simulink model "SR_SNN"  (R2022a)
settings: Solver=ode15s  StartTime=0.0  StopTime=NTimeSteps  RelTol=1e-3
values from neighbouring files (symbols this model uses):
  Etol = 10    [SR_Main_Script_Sim.m]
  t_iterO = 1    [SR_Main_Script_Sim.m]
  Ts = 1    [SR_Main_Script_Sim.m]
  Tx = 1    [SR_Main_Script_Sim.m]
  Txi = r*cos(xx)    [SR_Main_Script_Sim.m]
  Ty = 1    [SR_Main_Script_Sim.m]
  Tyi = r*sin(yy)    [SR_Main_Script_Sim.m]
  Tz = 2    [SR_Main_Script_Sim.m]
  x_i = [[1] ... (first row only)    [SR_Main_Script_Sim.m]
libraries: slpidlib x3, cstblocks x3, dspnetwork x2
settings Model: Creator=Pouya  LastModifiedBy=Pouya
settings DebuggingCC: UnconnectedInputMsg=warning  UnconnectedOutputMsg=warning  UnconnectedLineMsg=warning
settings RTWCC: DLArmComputeVersion=19.05

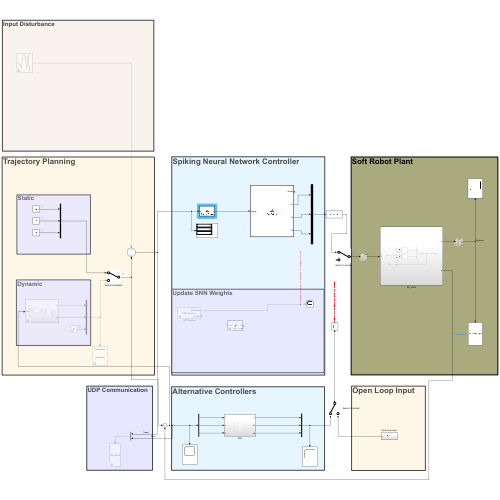
[thumbnail: Simulink's stored preview of the top-level diagram]
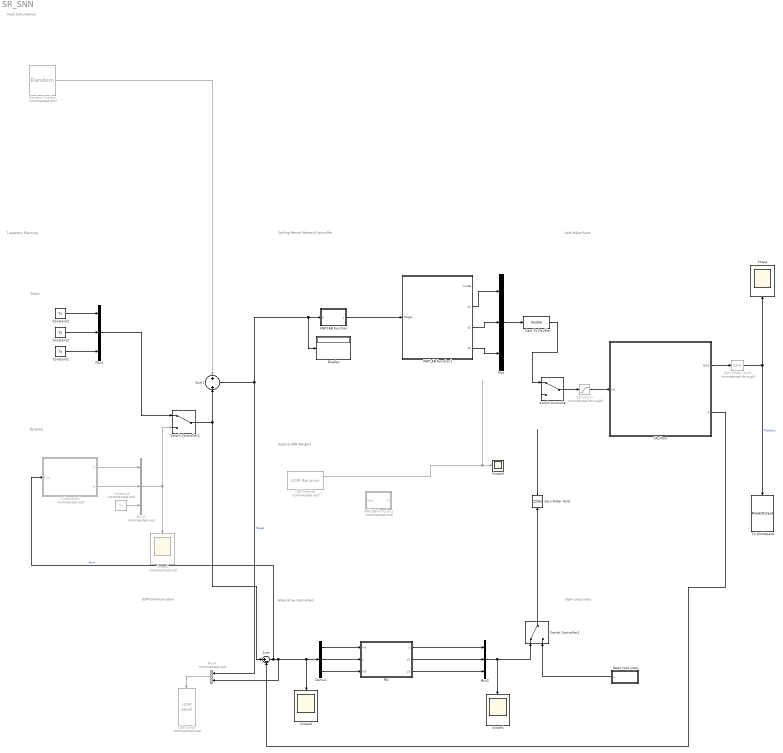
== system SR_SNN ==
  note: UDP Communication
  note: Update SNN Weights
  note: Input Disturbance
  note: Dynamic
  note: Static
  note: Open Loop Input
  note: Alternative Controllers
  note: Trajectory Planning
  note: Soft Robot Plant
  note: Spiking Neural Network Controller
  Cast To Double : DataTypeConversion  OutDataTypeStr=double  SaturateOnIntegerOverflow=off  RndMeth=Floor
  Constant1 : Constant  Value=Tz
  Constant2 : Constant  Value=Tx
  Constant3 : Constant  Value=Ty
  Constant4 : Constant  Commented=on  Value=Tz
  Demux : Demux  Outputs=3
  Display : Display
  MATLAB Function : MATLAB Function  TreatAsAtomicUnit=on
  MATLAB Function1 : MATLAB Function  TreatAsAtomicUnit=on
  MATLAB Function2 : MATLAB Function  Commented=on  TreatAsAtomicUnit=on
  Mux : Mux  Inputs=3
  Mux1 : Mux  Inputs=3
  Mux2 : Mux  Inputs=3
  Mux3 : Mux  Commented=on  Inputs=3
  Mux4 : Mux  Commented=on  Inputs=2
  Open loop input : Subsystem
  PID : Subsystem
  Random Number : RandomNumber  Commented=on  SampleTime=0.1
  SR_Plant : Subsystem
  Saturation : Saturate  Commented=through  UpperLimit=4  LowerLimit=-4
  Scope{,1,3..4} (4 alike) : Scope
  Scope2 : Scope  Commented=on
  Subsystem1 : Subsystem  Commented=on
  Sum : Sum  Inputs=|+-
  Sum1 : Sum
  Switch Controller : ManualSwitch
  Switch Controller1 : ManualSwitch
  Switch Controller2 : ManualSwitch
  To Workspace : ToWorkspace  VariableName=ModelOutput  SaveFormat=Timeseries  SampleTime=-1
  UDP Receive : dspnetwork/UDP Receive  Commented=on  localURL='0.0.0.0'  localPort=54320  remoteURL='127.0.0.1'  remotePort=-1  recvBufferSize=1024  dims=1  signalDatatype=uint8  isComplex=off  isVarSize=off  showBlockingTime=off  blockingTime=0  sampletime=1  blockPlatform=[]
  UDP Send1 : dspnetwork/UDP Send  Commented=on  remoteURL='127.0.0.1'  remotePort=54320  localURL='0.0.0.0'  localPortSource=Automatically determine  localPort=54320  sendBufferSize=1024  sampletime=-1  blockPlatform=[]  separateLengthPort=0
  Zero-Order Hold : ZeroOrderHold  SampleTime=Ts
  Zero-Order Hold1 : ZeroOrderHold  Commented=through  SampleTime=Ts
  wires:
  Constant2/1 -> Mux1/1
  Constant3/1 -> Mux1/2
  SR_Plant/1(Out1) -> Zero-Order Hold1/1
  SR_Plant/2(p) -> Sum/2
  Switch Controller/1 -> Saturation/1
  Constant1/1 -> Mux1/3
  Switch Controller1/1 -> Zero-Order Hold/1
  Open loop input/1(u) -> Switch Controller1/2
  Zero-Order Hold/1 -> ?
  Demux/2 -> PID/2(u)
  Demux/1 -> PID/1(In1)
  Demux/3 -> PID/3(In3)
  PID/1(y) -> Mux2/1
  Saturation/1 -> SR_Plant/1(In1)
  PID/2(y1) -> Mux2/2
  PID/3(y2) -> Mux2/3
  Mux2/1 -> Switch Controller1/1, Scope1/1
  Switch Controller2/1 -> Sum/1, Sum1/2
  Mux1/1 -> Switch Controller2/1
  Mux3/1 -> Switch Controller2/2, Scope2/1
  Subsystem1/2(Ty) -> Mux3/2
  Subsystem1/1(Tx) -> Mux3/1
  Constant4/1 -> Mux3/3
  MATLAB Function1/2(s1) -> Mux/1
  MATLAB Function1/3(s2) -> Mux/2
  MATLAB Function1/4(s3) -> Mux/3
  Sum/1 -> Scope3/1, Demux/1, Mux4/2, Subsystem1/1(Error)  "Error"
  Zero-Order Hold1/1 -> Scope/1, To Workspace/1  "Positions"
  UDP Receive/1 -> Scope4/1
  Random Number/1 -> Sum1/1
  Sum1/1 -> Display/1, MATLAB Function/1(u), Mux4/1  "Target"
  Mux4/1 -> UDP Send1/1
  MATLAB Function/1(y) -> MATLAB Function1/1(Target)
  Mux/1 -> Cast To Double/1
  Cast To Double/1 -> Switch Controller/1

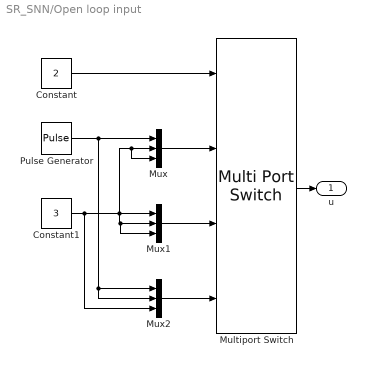
== system SR_SNN/Open loop input ==
  Constant : Constant  Value=2
  Constant1 : Constant  Value=3
  Multiport Switch : MultiPortSwitch  SaturateOnIntegerOverflow=off  InputSameDT=off
  Mux : Mux  Inputs=3
  Mux1 : Mux  Inputs=3
  Mux2 : Mux  Inputs=3
  Pulse Generator : DiscretePulseGenerator  PulseType=Time based  Period=5  PulseWidth=10
  u : Outport
  wires:
  Constant1/1 -> Mux2/3, Mux1/3, Mux1/2, Mux1/1, Mux/3, Mux/2
  Pulse Generator/1 -> Mux2/2, Mux2/1, Mux/1
  Constant/1 -> Multiport Switch/1
  Mux2/1 -> Multiport Switch/4
  Mux/1 -> Multiport Switch/2
  Multiport Switch/1 -> u/1
  Mux1/1 -> Multiport Switch/3

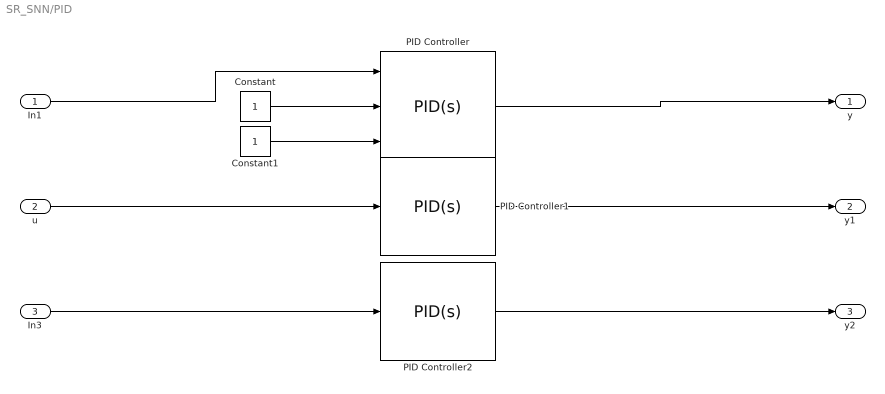
== system SR_SNN/PID ==
  In1 : Inport
  u : Inport  Port=2
  In3 : Inport  Port=3
  Constant : Constant
  Constant1 : Constant
  PID Controller : slpidlib/PID Controller  Controller=PID  Form=Parallel  TimeDomain=Continuous-time  UseExternalTs=off  SampleTime=-1  IntegratorMethod=Forward Euler  FilterMethod=Forward Euler  ControllerParametersSource=internal  P=-0.00389726842961966  I=-9.20575835453352e-05  UseKiTs=off  D=-0.0366591203292117  N=462.720758480725  UseFilter=on  TunerSelectOption=Transfer Function Based (PID Tuner App)  InitialConditionSource=external  InitialConditionForIntegrator=0  InitialConditionForFilter=0  DifferentiatorICPrevScaledInput=0  ExternalReset=none  TrackingMode=off  Kt=1  LimitOutput=off  SatLimitsSource=internal  UpperSaturationLimit=inf  LowerSaturationLimit=-inf  LinearizeAsGain=on  AntiWindupMode=none  Kb=1  POutMin=[]  POutMax=[]  IOutMin=[]  IOutMax=[]  DOutMin=[]  DOutMax=[]  NOutMin=[]  NOutMax=[]  SumOutMin=[]  SumOutMax=[]  SaturationOutMin=[]  SaturationOutMax=[]  PParamMin=[]  PParamMax=[]  IParamMin=[]  IParamMax=[]  DParamMin=[]  DParamMax=[]  NParamMin=[]  NParamMax=[]  KbParamMin=[]  KbParamMax=[]  KtParamMin=[]  KtParamMax=[]  KbOutMin=[]  KbOutMax=[]  KtOutMin=[]  KtOutMax=[]  IntegratorOutMin=[]  IntegratorOutMax=[]  FilterOutMin=[]  FilterOutMax=[]  SumI1OutMin=[]  SumI1OutMax=[]  SumI2OutMin=[]  SumI2OutMax=[]  SumI3OutMin=[]  SumI3OutMax=[]  SumI4OutMin=[]  SumI4OutMax=[]  SumDOutMin=[]  SumDOutMax=[]  DifferentiatorOutMin=[]  DifferentiatorOutMax=[]  FilterDiffOutCoefMin=[]  FilterDiffOutCoefMax=[]  ReciprocalOutMin=[]  ReciprocalOutMax=[]  SumDenOutMin=[]  SumDenOutMax=[]  SumNumOutMin=[]  SumNumOutMax=[]  DivideOutMin=[]  DivideOutMax=[]  UdiffTsProdOutMin=[]  UdiffTsProdOutMax=[]  NTsProdOutMin=[]  NTsProdOutMax=[]  UintegralTsProdOutMin=[]  UintegralTsProdOutMax=[]  UngainTsProdOutMin=[]  UngainTsProdOutMax=[]  IntegratorContinuousStateAttributes=''  IntegratorStateMustResolveToSignalObject=off  IntegratorRTWStateStorageClass=Auto  FilterContinuousStateAttributes=''  FilterStateMustResolveToSignalObject=off  FilterRTWStateStorageClass=Auto  ParallelPVariant=InternalParameters  IdealPVariant=Disabled  IVariant=InternalParameters  DVariant=InternalParameters  IntegratorVariant=Continuous  SatVariant=Disabled  AWVariant=Passthrough  PCopyVariant=Disabled  TRVariant=Disabled  FdbkBlocksVariant=Forward  IdealPFdbkVariant=Disabled  SatFdbkVariant=Disabled  DerivativeFilterVariant=ContFilter  NVariant=InternalParameters  NCopyVariant=Disabled  FilterICVariant=ExternalICs  IntegratorICVariant=ExternalICs  ExternalResetVariant=Disabled  TRSumVariant=Passthrough  SumFdbkVariant=Disabled  SumVariant=Sum_PID  TsampFilterVariant=InternalTs  TsampNgainVariant=Passthrough  TsampIntegralVariant=Passthrough  ExternalSaturationOutDataTypeStr=Inherit: Same as second input  aMode=0
  PID Controller1 : slpidlib/PID Controller  Controller=PID  Form=Parallel  TimeDomain=Continuous-time  UseExternalTs=off  SampleTime=-1  IntegratorMethod=Forward Euler  FilterMethod=Forward Euler  ControllerParametersSource=internal  P=0.79056648520257  I=12.0335076656055  UseKiTs=off  D=0.00902589117456867  N=93.9877255340492  UseFilter=on  TunerSelectOption=Transfer Function Based (PID Tuner App)  InitialConditionSource=internal  InitialConditionForIntegrator=0  InitialConditionForFilter=0  DifferentiatorICPrevScaledInput=0  ExternalReset=none  TrackingMode=off  Kt=1  LimitOutput=off  SatLimitsSource=internal  UpperSaturationLimit=inf  LowerSaturationLimit=-inf  LinearizeAsGain=on  AntiWindupMode=none  Kb=1  POutMin=[]  POutMax=[]  IOutMin=[]  IOutMax=[]  DOutMin=[]  DOutMax=[]  NOutMin=[]  NOutMax=[]  SumOutMin=[]  SumOutMax=[]  SaturationOutMin=[]  SaturationOutMax=[]  PParamMin=[]  PParamMax=[]  IParamMin=[]  IParamMax=[]  DParamMin=[]  DParamMax=[]  NParamMin=[]  NParamMax=[]  KbParamMin=[]  KbParamMax=[]  KtParamMin=[]  KtParamMax=[]  KbOutMin=[]  KbOutMax=[]  KtOutMin=[]  KtOutMax=[]  IntegratorOutMin=[]  IntegratorOutMax=[]  FilterOutMin=[]  FilterOutMax=[]  SumI1OutMin=[]  SumI1OutMax=[]  SumI2OutMin=[]  SumI2OutMax=[]  SumI3OutMin=[]  SumI3OutMax=[]  SumI4OutMin=[]  SumI4OutMax=[]  SumDOutMin=[]  SumDOutMax=[]  DifferentiatorOutMin=[]  DifferentiatorOutMax=[]  FilterDiffOutCoefMin=[]  FilterDiffOutCoefMax=[]  ReciprocalOutMin=[]  ReciprocalOutMax=[]  SumDenOutMin=[]  SumDenOutMax=[]  SumNumOutMin=[]  SumNumOutMax=[]  DivideOutMin=[]  DivideOutMax=[]  UdiffTsProdOutMin=[]  UdiffTsProdOutMax=[]  NTsProdOutMin=[]  NTsProdOutMax=[]  UintegralTsProdOutMin=[]  UintegralTsProdOutMax=[]  UngainTsProdOutMin=[]  UngainTsProdOutMax=[]  IntegratorContinuousStateAttributes=''  IntegratorStateMustResolveToSignalObject=off  IntegratorRTWStateStorageClass=Auto  FilterContinuousStateAttributes=''  FilterStateMustResolveToSignalObject=off  FilterRTWStateStorageClass=Auto  ParallelPVariant=InternalParameters  IdealPVariant=Disabled  IVariant=InternalParameters  DVariant=InternalParameters  IntegratorVariant=Continuous  SatVariant=Disabled  AWVariant=Passthrough  PCopyVariant=Disabled  TRVariant=Disabled  FdbkBlocksVariant=Forward  IdealPFdbkVariant=Disabled  SatFdbkVariant=Disabled  DerivativeFilterVariant=ContFilter  NVariant=InternalParameters  NCopyVariant=Disabled  FilterICVariant=InternalICsFilter  IntegratorICVariant=InternalICs  ExternalResetVariant=Disabled  TRSumVariant=Passthrough  SumFdbkVariant=Disabled  SumVariant=Sum_PID  TsampFilterVariant=InternalTs  TsampNgainVariant=Passthrough  TsampIntegralVariant=Passthrough  ExternalSaturationOutDataTypeStr=Inherit: Same as second input  aMode=0
  PID Controller2 : slpidlib/PID Controller  Controller=PID  Form=Parallel  TimeDomain=Continuous-time  UseExternalTs=off  SampleTime=-1  IntegratorMethod=Forward Euler  FilterMethod=Forward Euler  ControllerParametersSource=internal  P=0.559243071667532  I=12.7287987560963  UseKiTs=off  D=0  N=100  UseFilter=on  TunerSelectOption=Transfer Function Based (PID Tuner App)  InitialConditionSource=internal  InitialConditionForIntegrator=0  InitialConditionForFilter=0  DifferentiatorICPrevScaledInput=0  ExternalReset=none  TrackingMode=off  Kt=1  LimitOutput=off  SatLimitsSource=internal  UpperSaturationLimit=inf  LowerSaturationLimit=-inf  LinearizeAsGain=on  AntiWindupMode=none  Kb=1  POutMin=[]  POutMax=[]  IOutMin=[]  IOutMax=[]  DOutMin=[]  DOutMax=[]  NOutMin=[]  NOutMax=[]  SumOutMin=[]  SumOutMax=[]  SaturationOutMin=[]  SaturationOutMax=[]  PParamMin=[]  PParamMax=[]  IParamMin=[]  IParamMax=[]  DParamMin=[]  DParamMax=[]  NParamMin=[]  NParamMax=[]  KbParamMin=[]  KbParamMax=[]  KtParamMin=[]  KtParamMax=[]  KbOutMin=[]  KbOutMax=[]  KtOutMin=[]  KtOutMax=[]  IntegratorOutMin=[]  IntegratorOutMax=[]  FilterOutMin=[]  FilterOutMax=[]  SumI1OutMin=[]  SumI1OutMax=[]  SumI2OutMin=[]  SumI2OutMax=[]  SumI3OutMin=[]  SumI3OutMax=[]  SumI4OutMin=[]  SumI4OutMax=[]  SumDOutMin=[]  SumDOutMax=[]  DifferentiatorOutMin=[]  DifferentiatorOutMax=[]  FilterDiffOutCoefMin=[]  FilterDiffOutCoefMax=[]  ReciprocalOutMin=[]  ReciprocalOutMax=[]  SumDenOutMin=[]  SumDenOutMax=[]  SumNumOutMin=[]  SumNumOutMax=[]  DivideOutMin=[]  DivideOutMax=[]  UdiffTsProdOutMin=[]  UdiffTsProdOutMax=[]  NTsProdOutMin=[]  NTsProdOutMax=[]  UintegralTsProdOutMin=[]  UintegralTsProdOutMax=[]  UngainTsProdOutMin=[]  UngainTsProdOutMax=[]  IntegratorContinuousStateAttributes=''  IntegratorStateMustResolveToSignalObject=off  IntegratorRTWStateStorageClass=Auto  FilterContinuousStateAttributes=''  FilterStateMustResolveToSignalObject=off  FilterRTWStateStorageClass=Auto  ParallelPVariant=InternalParameters  IdealPVariant=Disabled  IVariant=InternalParameters  DVariant=InternalParameters  IntegratorVariant=Continuous  SatVariant=Disabled  AWVariant=Passthrough  PCopyVariant=Disabled  TRVariant=Disabled  FdbkBlocksVariant=Forward  IdealPFdbkVariant=Disabled  SatFdbkVariant=Disabled  DerivativeFilterVariant=ContFilter  NVariant=InternalParameters  NCopyVariant=Disabled  FilterICVariant=InternalICsFilter  IntegratorICVariant=InternalICs  ExternalResetVariant=Disabled  TRSumVariant=Passthrough  SumFdbkVariant=Disabled  SumVariant=Sum_PID  TsampFilterVariant=InternalTs  TsampNgainVariant=Passthrough  TsampIntegralVariant=Passthrough  ExternalSaturationOutDataTypeStr=Inherit: Same as second input  aMode=0
  y : Outport
  y1 : Outport  Port=2
  y2 : Outport  Port=3
  wires:
  u/1 -> PID Controller1/1
  PID Controller/1 -> y/1
  In1/1 -> PID Controller/1
  PID Controller1/1 -> y1/1
  In3/1 -> PID Controller2/1
  PID Controller2/1 -> y2/1
  Constant/1 -> PID Controller/2
  Constant1/1 -> PID Controller/3

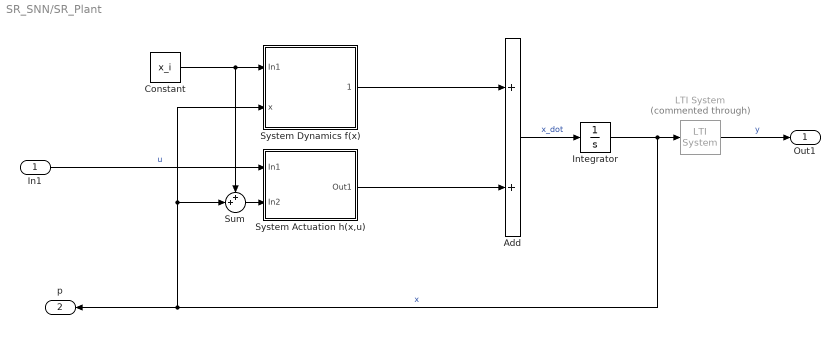
== system SR_SNN/SR_Plant ==
  In1 : Inport
  Add : Sum
  Constant : Constant  Value=x_i
  Integrator : Integrator
  LTI System : cstblocks/LTI System  Commented=through  sys=C  IC=[]
  Sum : Sum  Inputs=++|
  System Actuation h(x,u) : Subsystem
  System Dynamics f(x) : Subsystem
  Out1 : Outport
  p : Outport  Port=2
  wires:
  In1/1 -> System Actuation h(x,u)/1(In1)  "u"
  System Dynamics f(x)/1(1) -> Add/1
  System Actuation h(x,u)/1(Out1) -> Add/2
  Add/1 -> Integrator/1  "x_dot"
  Constant/1 -> Sum/1, System Dynamics f(x)/1(In1)
  Integrator/1 -> System Dynamics f(x)/2(x), Sum/2, p/1, LTI System/1  "x"
  LTI System/1 -> Out1/1  "y"
  Sum/1 -> System Actuation h(x,u)/2(In2)

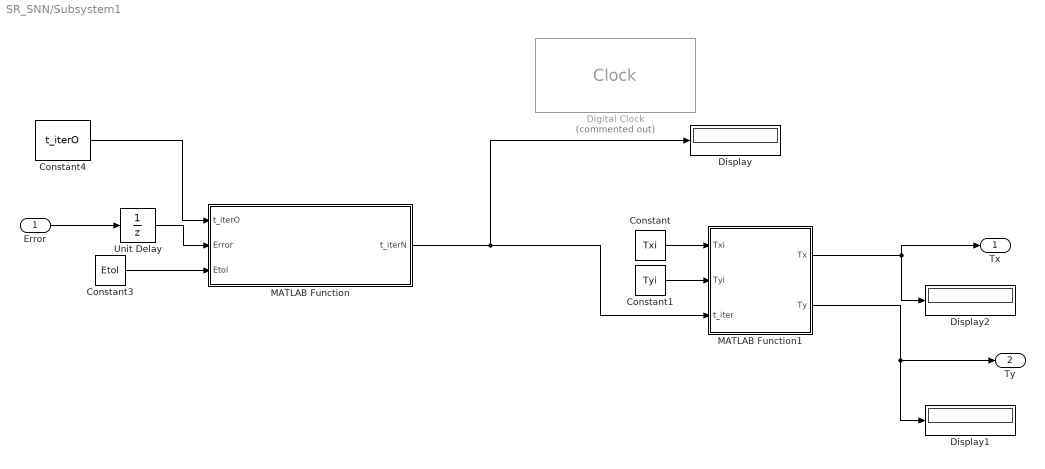
== system SR_SNN/Subsystem1 ==
  Error : Inport
  Constant : Constant  Value=Txi
  Constant1 : Constant  Value=Tyi
  Constant3 : Constant  Value=Etol
  Constant4 : Constant  Value=t_iterO
  Digital Clock : DigitalClock  Commented=on
  Display : Display
  Display1 : Display
  Display2 : Display
  MATLAB Function : MATLAB Function  TreatAsAtomicUnit=on
  MATLAB Function1 : MATLAB Function  TreatAsAtomicUnit=on
  Unit Delay : UnitDelay  SampleTime=-1  HasFrameUpgradeWarning=on
  Tx : Outport
  Ty : Outport  Port=2
  wires:
  MATLAB Function1/1(Tx) -> Tx/1, Display2/1
  MATLAB Function1/2(Ty) -> Display1/1, Ty/1
  Error/1 -> Unit Delay/1
  Constant3/1 -> MATLAB Function/3(Etol)
  MATLAB Function/1(t_iterN) -> Display/1, MATLAB Function1/3(t_iter)
  Unit Delay/1 -> MATLAB Function/2(Error)
  Constant4/1 -> MATLAB Function/1(t_iterO)
  Constant1/1 -> MATLAB Function1/2(Tyi)
  Constant/1 -> MATLAB Function1/1(Txi)

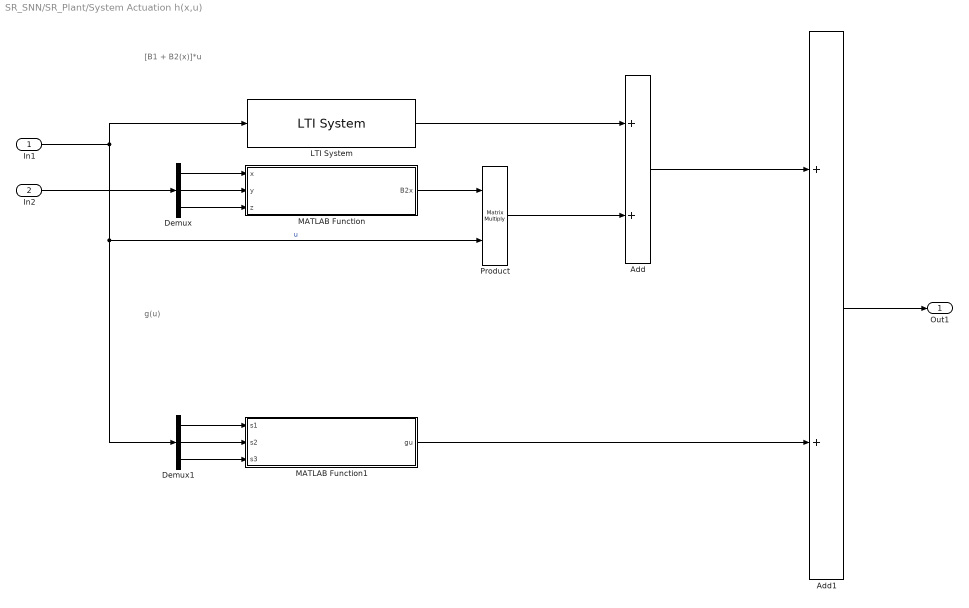
== system SR_SNN/SR_Plant/System Actuation h(x,u) ==
  note: g(u)
  note: [B1 + B2(x)]*u
  In1 : Inport
  In2 : Inport  Port=2
  Add : Sum
  Add1 : Sum
  Demux : Demux  Outputs=3
  Demux1 : Demux  Outputs=3
  LTI System : cstblocks/LTI System  sys=B1  IC=[]
  MATLAB Function : MATLAB Function  TreatAsAtomicUnit=on
  MATLAB Function1 : MATLAB Function  TreatAsAtomicUnit=on
  Product : Product  Multiplication=Matrix(*)
  Out1 : Outport
  wires:
  In1/1 -> LTI System/1, Demux1/1, Product/2  "u"
  MATLAB Function1/1(gu) -> Add1/2
  LTI System/1 -> Add/1
  Product/1 -> Add/2
  Add/1 -> Add1/1
  MATLAB Function/1(B2x) -> Product/1
  Add1/1 -> Out1/1
  In2/1 -> Demux/1
  Demux/2 -> MATLAB Function/2(y)
  Demux/1 -> MATLAB Function/1(x)
  Demux/3 -> MATLAB Function/3(z)
  Demux1/2 -> MATLAB Function1/2(s2)
  Demux1/1 -> MATLAB Function1/1(s1)
  Demux1/3 -> MATLAB Function1/3(s3)

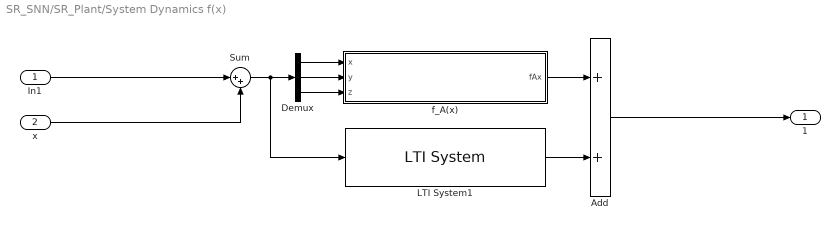
== system SR_SNN/SR_Plant/System Dynamics f(x) ==
  In1 : Inport
  x : Inport  Port=2
  Add : Sum
  Demux : Demux  Outputs=3
  LTI System1 : cstblocks/LTI System  sys=A  IC=[]
  Sum : Sum  Inputs=|++
  f_A(x) : MATLAB Function  TreatAsAtomicUnit=on
  1 : Outport
  wires:
  In1/1 -> Sum/1
  Sum/1 -> LTI System1/1, Demux/1
  Add/1 -> 1/1
  LTI System1/1 -> Add/2
  f_A(x)/1(fAx) -> Add/1
  Demux/1 -> f_A(x)/1(x)
  Demux/2 -> f_A(x)/2(y)
  Demux/3 -> f_A(x)/3(z)
  x/1 -> Sum/2

== matlab function SR_SNN/MATLAB Function1 ==
  data: model output; s1 output; s2 output; s3 output; Target input
 function [model,s1,s2,s3] = RunPython(Target)
    model=0;s1=0;s2=0;s3=0;% Has to be preassigned, otherwise Simulink throws an error
    coder.extrinsic('py.SNN_model.Run_model') % Python functions have to be run extrinsically, meaning no C code generated
    [model,s1,s2,s3] = py.SNN_model.Run_model(Target);
    
end

== matlab function SR_SNN/SR_Plant/System Dynamics f(x)/f_A(x) ==
  data: x input; fAx output; y input; z input
function fAx = f_A(x,y,z)

fAx = 10e-3*[[0.17*x^2 - 1.22*y^2 - 0.145*z^2 + 4.92*x*y + 20.3*x*z + 0.748*y*z]
           [3.39*x^2 - 1.94*y^2 + 3.48*z^2 - 1.68*x*y + 5.63*x*z + 17.0*y*z]
           [0.456*x^2 + 0.672*y^2 + 19.4*z^2 - 1.92*x*y + 1.3*x*z - 0.0985*y*z]];

== matlab function SR_SNN/SR_Plant/System Actuation h(x,u)/MATLAB Function ==
  data: x input; B2x output; y input; z input
function B2x = B2(x,y,z)

B2x = 10e-3*[[-2.86*x + 2.34*y + 16.8*z, -2.56*x - 1.23*y - 20.2*z, 1.59*x - 1.16*y + 3.61*z]
             [2.76*x + 0.356*y - 9.28*z, -2.98*x + 3.22*y - 12.9*z, -0.129*x - 4.02*y + 19.9*z]
             [-4.72*x + 3.42*y + 2.26*z, 5.47*x + 3.28*y + 1.58*z, -1.06*x - 6.62*y + 4.49*z]];

== matlab function SR_SNN/SR_Plant/System Actuation h(x,u)/MATLAB Function1 ==
  data: s1 input; gu output; s2 input; s3 input
function gu = g(s1,s2,s3)

gu = 10e-4*[[14.1*s1^2 - 8.48*s2^2 + 5.9*s3^2 - 5.02*s1*s2 - 6.56*s1*s3 + 3.04*s2*s3]
            [11.3*s1^2 - 4.67*s2^2 + 19.5*s3^2 + 1.54*s1*s2 + 3.15*s1*s3 - 1.25*s2*s3]
            [1.05*s1^2 + 2.26*s2^2 + 2.83*s3^2 - 10.6*s1*s2 - 3.2*s1*s3 - 12.7*s2*s3]];

== matlab function SR_SNN/MATLAB Function ==
  data: u input; y output
function y = ConvertDtype(u)

y = 0;
coder.extrinsic('Mat2Py')
y = Mat2Py(u);

== matlab function SR_SNN/Subsystem1/MATLAB Function ==
  data: t_iterO input; Error input; t_iterN output; Etol input
function t_iterN = Target_hit(t_iterO,Error,Etol)

if norm(Error) < Etol
    t_iterN = t_iterO+1;
%     t_iterO = t_iterN;

else
    t_iterN = t_iterO;
end
end

== matlab function SR_SNN/Subsystem1/MATLAB Function1 ==
  data: Txi input; Tx output; Tyi input; t_iter input; Ty output
function [Tx,Ty] = TargetSelector(Txi,Tyi,t_iter)

Tx = Txi(t_iter);
Ty = Tyi(t_iter);

end

== matlab function SR_SNN/MATLAB Function2 ==
  data: Error input; W output
function W = UpdateSNNWeights(Error)
  W=0;% Has to be preassigned, otherwise Simulink throws an error
  coder.extrinsic('py.SNN_model') % Python functions have to be run extrinsically, meaning no C code generated
  W = py.SNN_model.Update(Error);
